simulink model "two_tanks_tracking_controller_1"  (R2021b)
settings: Solver=ode5  StartTime=0.0  StopTime=150  FixedStep=0.1  RelTol=1e-3  EnableMultiTasking=on
values from neighbouring files (symbols this model uses):
  A = -1    [estimator.m]    (also in main_quad.m = jacobian(1:12,1:12); two_tanks_tracking_controller.m = [-0.0891 0.0891)
  B = 1    [estimator.m]    (also in main_quad.m = jacobian(1:12,13:16); two_tanks_tracking_controller.m = [14.0845 0)
  C = 1    [estimator.m]    (also in main_quad.m = [eye(3) zeros(3,9); two_tanks_tracking_controller.m = [1 0)
  K = place(A,B,cl_poles)    [two_tanks_tracking_controller.m]
  Nu = big_N(nx+1:end,:)    [main_quad.m]    (also in two_tanks_tracking_controller.m = big_N (nx+1:end,:))
  Nx = big_N(1:nx,:)    [main_quad.m]    (also in two_tanks_tracking_controller.m)
settings Model: Creator=magudelo  LastModifiedBy=ludvig
settings SolverCC: AlgebraicLoopSolver=TrustRegion
settings DataIOCC: SaveFormat=Array  SignalLoggingSaveFormat=ModelDataLogs  ReturnWorkspaceOutputs=off
settings OptimizationCC: BlockReduction=off  BooleanDataType=off  ExpressionDepthLimit=2147483647  LifeSpan=inf
settings DebuggingCC: SaveWithParameterizedLinksMsg=none  UnderspecifiedInitializationDetection=Classic  MergeDetectMultiDrivingBlocksExec=none  SignalResolutionControl=TryResolveAllWithWarning  MultiTaskDSMMsg=warning  MultiTaskCondExecSysMsg=none  FcnCallInpInsideContextMsg=warning  AllowSymbolicDim=off  StateNameClashWarn=warning  SFUnexpectedBacktrackingDiag=warning  SFNoUnconditionalDefaultTransitionDiag=warning  SFExecutionAtInitializationDiag=none  SFMachineParentedDataDiag=warning  ArithmeticOperatorsInVariantConditions=warning
settings HardwareCC: ProdBitPerPointer=32  ProdBitPerSizeT=32  ProdBitPerPtrDiffT=32  ProdLargestAtomicFloat=None  ProdIntDivRoundTo=Undefined  ProdEndianess=Unspecified  ProdWordSize=32  ProdHWDeviceType=32-bit Generic  TargetUnknown=on
settings ModelReferenceCC: PropagateSignalLabelsOutOfModel=off
settings SFSimCC: SimUseLocalCustomCode=off  CustomCodeUndefinedFunction=UseInterfaceOnly
settings RTWCC: RTWUseLocalCustomCode=off
settings CodeAppCC: StateflowObjectComments=on
settings GRTTargetCC: TargetLangStandard=C89/C90 (ANSI)  CombineOutputUpdateFcns=off  GRTInterface=on
settings ConfigComp: CovMetricSettings=dw  CovSaveCumulativeToWorkspaceVar=on  CovSaveSingleToWorkspaceVar=on  CovExternalEMLEnable=off

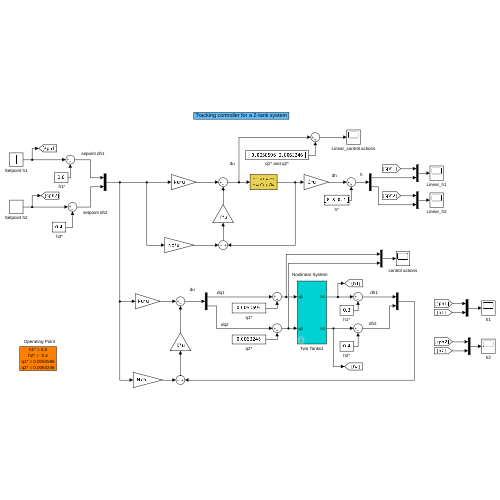
[thumbnail: Simulink's stored preview of the top-level diagram]
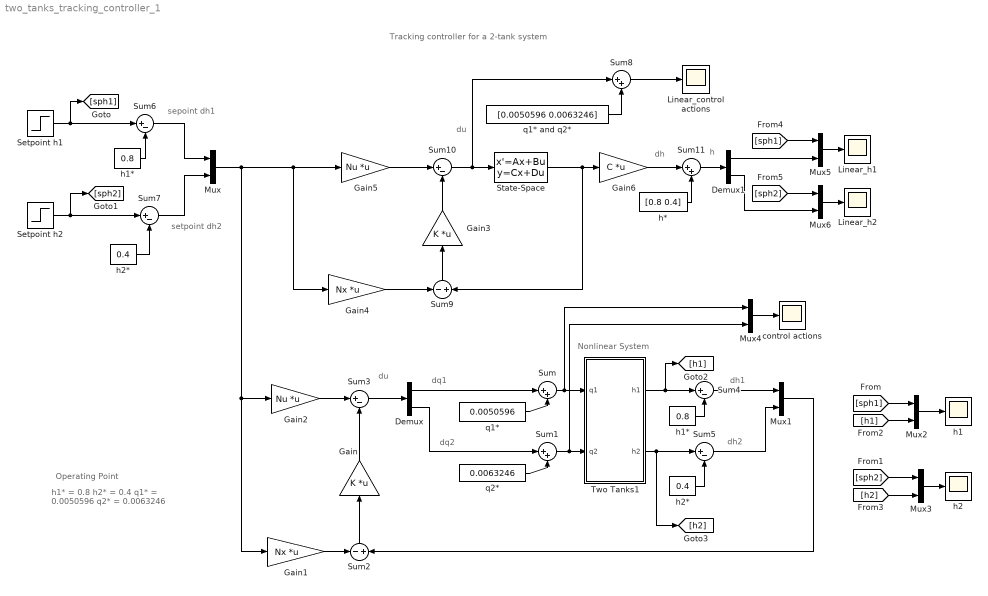
== system two_tanks_tracking_controller_1 ==
  note: h
  note: du
  note: Nonlinear System
  note: Tracking controller for a 2-tank system
  note: Operating Point
  note: h1* = 0.8
      | h2* =  0.4
      | q1* = 0.0050596
      | q2* = 0.0063246
  note: dh1
  note: dh2
  note: dq1
  note: dq2
  note: sepoint dh1
  note: setpoint dh2
  note: dh
  note: du
  " h1*" : Constant  Value=0.8
  " h2*" : Constant  Value=0.4
  Demux : Demux  Outputs=2
  Demux1 : Demux  Outputs=2
  Gain : Gain  Gain=K  Multiplication=Matrix(K*u)
  Gain1 : Gain  Gain=Nx  Multiplication=Matrix(K*u)
  Gain2 : Gain  Gain=Nu  Multiplication=Matrix(K*u)
  Gain3 : Gain  Gain=K  Multiplication=Matrix(K*u)
  Gain4 : Gain  Gain=Nx  Multiplication=Matrix(K*u)
  Gain5 : Gain  Gain=Nu  Multiplication=Matrix(K*u)
  Gain6 : Gain  Gain=C  Multiplication=Matrix(K*u)
  Linear_control actions : Scope
  Linear_h1 : Scope
  Linear_h2 : Scope
  Mux{,1..6} (7 alike) : Mux  Inputs=2
  Setpoint h1 : Step  Time=50  Before=0.8  After=0.9  SampleTime=0
  Setpoint h2 : Step  Time=50  Before=0.4  After=0.4  SampleTime=0
  State-Space : StateSpace  A=A  B=B  C=eye(2,2)  D=zeros(2,2)  InitialCondition=0
  Sum{,1,8,11} (4 alike) : Sum  Inputs=|++  InputSameDT=on  SaturateOnIntegerOverflow=on  OutDataTypeStr=Inherit: Same as first input
  Sum{3..7,10} (6 alike) : Sum  Inputs=|+-  InputSameDT=on  SaturateOnIntegerOverflow=on  OutDataTypeStr=Inherit: Same as first input
  Sum2 : Sum  Inputs=-+  InputSameDT=on  SaturateOnIntegerOverflow=on  OutDataTypeStr=Inherit: Same as first input
  Sum9 : Sum  Inputs=-+  InputSameDT=on  SaturateOnIntegerOverflow=on  OutDataTypeStr=Inherit: Same as first input
  Two Tanks1 : Subsystem  mask(Tanks systems){A1=0.071, A2=0.071, k1=0.008, k2=0.018, h10=0.8, h20=0.4}
      mask prompts: A1 "Cross sectional area of Tank 1 :"; A2 "Cross sectional area of Tank 2  :"; k1 "Valve coefficient k1 :"; k2 "Valve coeficient k2 :"; h10 "Initial level for Tank 1:"; h20 "Initial level for Tank 2 :"
      mask help:
      | Sistema de 2 tanques acoplados.
      |
      | Oscar Mauricio Agudelo Mañozca
      | OMAM/2002
  control actions : Scope
  h* : Constant  Value=[0.8 0.4]
  h1 : Scope
  h1* : Constant  Value=0.8
  h2 : Scope
  h2* : Constant  Value=0.4
  q1* : Constant  Value=0.0050596
  q1* and q2* : Constant  Value=[0.0050596 0.0063246]
  q2* : Constant  Value=0.0063246
  wires:
  Sum/1 -> Two Tanks1/1(q1), Mux4/1
  q1*/1 -> Sum/2
  Sum1/1 -> Two Tanks1/2(q2), Mux4/2
  q2*/1 -> Sum1/2
  Two Tanks1/1(h1) -> Sum4/1, [h1]
  h1*/1 -> Sum4/2
  h2*/1 -> Sum5/2
  Two Tanks1/2(h2) -> Sum5/1, [h2]
  Sum4/1 -> Mux1/1
  Sum5/1 -> Mux1/2
  Mux1/1 -> Sum2/2
  Sum2/1 -> Gain/1
  Gain1/1 -> Sum2/1
  Mux/1 -> Gain2/1, Gain1/1, Gain5/1, Gain4/1
  Gain2/1 -> Sum3/1
  Gain/1 -> Sum3/2
  Sum3/1 -> Demux/1
  Demux/1 -> Sum/1
  Demux/2 -> Sum1/1
  Setpoint h1/1 -> Sum6/1, [sph1]
  " h1*"/1 -> Sum6/2
  Setpoint h2/1 -> Sum7/1, [sph2]
  " h2*"/1 -> Sum7/2
  Sum7/1 -> Mux/2
  Sum6/1 -> Mux/1
  Mux2/1 -> h1/1
  Mux3/1 -> h2/1
  [sph1] -> Mux2/1
  [sph2] -> Mux3/1
  [h1] -> Mux2/2
  [h2] -> Mux3/2
  Mux4/1 -> control actions/1
  Sum9/1 -> Gain3/1
  Gain4/1 -> Sum9/1
  Gain5/1 -> Sum10/1
  Gain3/1 -> Sum10/2
  Sum10/1 -> State-Space/1, Sum8/1
  Mux5/1 -> Linear_h1/1
  Mux6/1 -> Linear_h2/1
  [sph1] -> Mux5/1
  [sph2] -> Mux6/1
  Demux1/1 -> Mux5/2
  State-Space/1 -> Gain6/1, Sum9/2
  Gain6/1 -> Sum11/1
  h*/1 -> Sum11/2
  Sum11/1 -> Demux1/1
  Demux1/2 -> Mux6/2
  q1* and q2*/1 -> Sum8/2
  Sum8/1 -> Linear_control actions/1

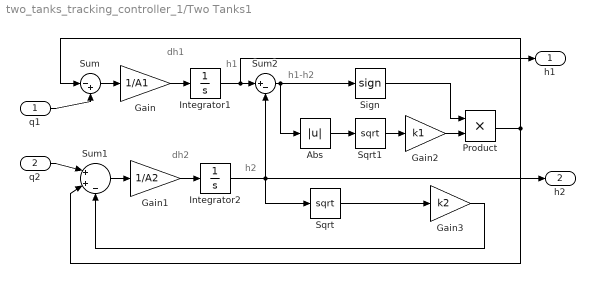
== system two_tanks_tracking_controller_1/Two Tanks1 ==
  note: h1-h2
  note: h2
  note: dh2
  note: h1
  note: dh1
  q1 : Inport
  q2 : Inport  Port=2
  Abs : Abs  SaturateOnIntegerOverflow=on
  Gain : Gain  Gain=1/A1  SaturateOnIntegerOverflow=on  OutDataTypeStr=Inherit: Same as input  ParamDataTypeStr=Inherit: Same as input
  Gain1 : Gain  Gain=1/A2  SaturateOnIntegerOverflow=on  OutDataTypeStr=Inherit: Same as input  ParamDataTypeStr=Inherit: Same as input
  Gain2 : Gain  Gain=k1  SaturateOnIntegerOverflow=on  OutDataTypeStr=Inherit: Same as input  ParamDataTypeStr=Inherit: Same as input
  Gain3 : Gain  Gain=k2  SaturateOnIntegerOverflow=on  OutDataTypeStr=Inherit: Same as input  ParamDataTypeStr=Inherit: Same as input
  Integrator1 : Integrator  InitialCondition=h10  LimitOutput=on  LowerSaturationLimit=0
  Integrator2 : Integrator  InitialCondition=h20  LimitOutput=on  LowerSaturationLimit=0
  Product : Product  InputSameDT=on  RndMeth=Zero  SaturateOnIntegerOverflow=on  OutDataTypeStr=Inherit: Same as first input
  Sign : Signum
  Sqrt : Sqrt  SaturateOnIntegerOverflow=on
  Sqrt1 : Sqrt  SaturateOnIntegerOverflow=on
  Sum : Sum  Inputs=|-+  InputSameDT=on  SaturateOnIntegerOverflow=on  OutDataTypeStr=Inherit: Same as first input
  Sum1 : Sum  Inputs=|++-  InputSameDT=on  SaturateOnIntegerOverflow=on  OutDataTypeStr=Inherit: Same as first input
  Sum2 : Sum  Inputs=|+-  InputSameDT=on  SaturateOnIntegerOverflow=on  OutDataTypeStr=Inherit: Same as first input
  h1 : Outport
  h2 : Outport  Port=2
  wires:
  Sum/1 -> Gain/1
  Gain/1 -> Integrator1/1
  Product/1 -> Sum/1, Sum1/2
  Integrator1/1 -> Sum2/1, h1/1
  q1/1 -> Sum/2
  Sum2/1 -> Abs/1, Sign/1
  Abs/1 -> Sqrt1/1
  Sqrt1/1 -> Gain2/1
  Gain2/1 -> Product/2
  Sign/1 -> Product/1
  Sum1/1 -> Gain1/1
  Gain1/1 -> Integrator2/1
  q2/1 -> Sum1/1
  Gain3/1 -> Sum1/3
  Integrator2/1 -> Sqrt/1, Sum2/2, h2/1
  Sqrt/1 -> Gain3/1
